simulink model "Acc_Interface"  (R2024b)
settings: Solver=FixedStepAuto  StartTime=0.0  StopTime=inf  FixedStep=5e-3  RelTol=1e-3
InitFcn:
  | %run('config.m');
libraries: arduinolib x2
settings Model: ExtModeTrigDuration=2  Creator=Marc  LastModifiedBy=Nitesh
settings SolverCC: AutoInsertRateTranBlk=on
settings OptimizationCC: DefaultParameterBehavior=Inlined  GainParamInheritBuiltInType=on  UseFloatMulNetSlope=on  InlineInvariantSignals=on  EnhancedBackFolding=on  PassReuseOutputArgsAs=Individual arguments  ZeroExternalMemoryAtStartup=off  ZeroInternalMemoryAtStartup=off  EfficientFloat2IntCast=on  MaxStackSize=64  OptimizeBlockOrder=speed  DifferentSizesBufferReuse=on  OptimizationCustomize=off  EfficientTunableParamExpr=on
settings DebuggingCC: SaveWithParameterizedLinksMsg=none  UnderspecifiedInitializationDetection=Classic  MergeDetectMultiDrivingBlocksExec=none  SignalResolutionControl=TryResolveAllWithWarning  ParameterTunabilityLossMsg=error
settings HardwareCC: ProdBitPerPointer=32  ProdBitPerSizeT=32  ProdBitPerPtrDiffT=32  ProdLargestAtomicInteger=Long  ProdLargestAtomicFloat=Double  ProdWordSize=32  ProdHWDeviceType=ARM Compatible->ARM Cortex  TargetIntDivRoundTo=Zero  TargetEndianess=LittleEndian  TargetHWDeviceType=Custom Processor->Custom Processor  ProdEqTarget=off  UseEmbeddedCoderFeatures=off
settings ModelReferenceCC: PropagateSignalLabelsOutOfModel=off
settings RTWCC: Description=Embedded Coder  SystemTargetFile=ert.tlc  HardwareBoard=ESP32-WROOM(Arduino Compatible)  TLCOptions="-aInlineSetEventsForThisBaseRateFcn=TLC_FALSE -aSuppressMultiTaskScheduler=TLC_FALSE  -aRateBasedStepFcn=0"  TemplateMakefile=ert_default_tmf  Toolchain=ESP32  BuildConfiguration=Faster Runs
settings CodeAppCC: ForceParamTrailComments=on  IgnoreCustomStorageClasses=off  OperatorAnnotations=on  SimulinkDataObjDesc=on  SFDataObjDesc=on  InsertBlockDesc=on
settings ERTTargetCC: SupportNonFinite=off  SupportContinuousTime=on  SupportNonInlinedSFcns=on  SupportVariableSizeSignals=on  ExtModeTransport=3  ExtModeStaticAlloc=on  ExtModeAutomaticAllocSize=off  ExtModeStaticAllocSize=65536  ExtModeMexFile=ext_xcp  ExtModeIntrfLevel=Level2 - Open  InlinedParameterPlacement=Hierarchical

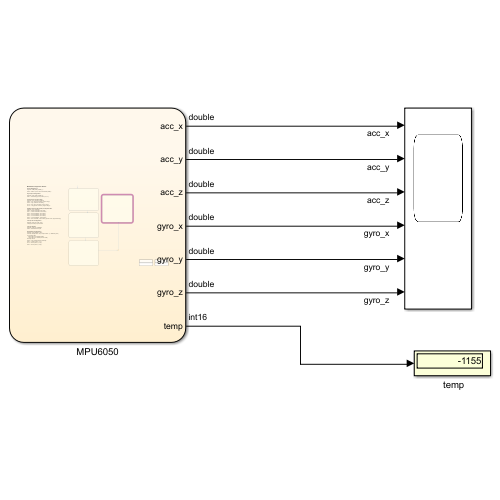
[thumbnail: Simulink's stored preview of the top-level diagram]
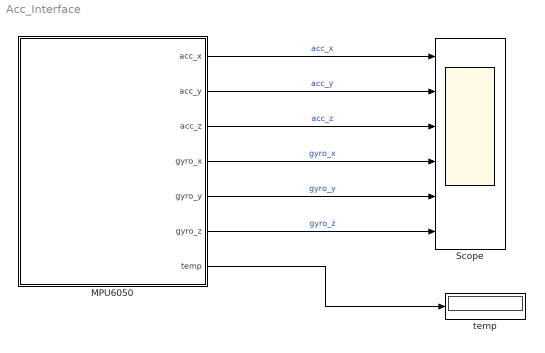
== system Acc_Interface ==
  " temp" : Display
  MPU6050 : Stateflow chart  TreatAsAtomicUnit=on
  Scope : Scope  NumInputPorts=6
  wires:
  MPU6050/1(acc_x) -> Scope/1  "acc_x"
  MPU6050/2(acc_y) -> Scope/2  "acc_y"
  MPU6050/3(acc_z) -> Scope/3  "acc_z"
  MPU6050/7(temp) -> " temp"/1
  MPU6050/4(gyro_x) -> Scope/4  "gyro_x"
  MPU6050/5(gyro_y) -> Scope/5  "gyro_y"
  MPU6050/6(gyro_z) -> Scope/6  "gyro_z"

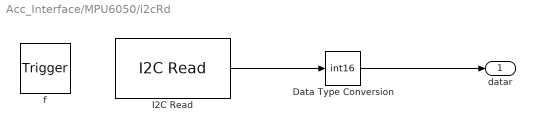
== system Acc_Interface/MPU6050/i2cRd ==
  f : TriggerPort  TriggerType=function-call  VariantControl=Variant  SampleTime=inf
      settings: CopyFcn=Stateflow.SLINSF.SimulinkMan.removeBlockPreDeleteFcn  PreDeleteFcn=Stateflow.SLINSF.SimulinkMan.unsafePredeleteFcn
  Data Type Conversion : DataTypeConversion  OutDataTypeStr=int16  SaturateOnIntegerOverflow=off  RndMeth=Floor
  I2C Read : arduinolib/I2C Read  I2CModule=0  Mode=Master  SlaveAddress=hex2dec( '68' )  SlaveByteOrder=BigEndian  Direction=Receiver  RegisterAddressMode=on  RegisterAddress=hex2dec( '3b' )  SlaveDataType=uint16  DataLength=7  NoAck=off  RepeatedStart=off  OutputStatus=off  blockPlatform=arduino  SampleTime=-1
      settings: SourceProductName=Common
  datar : Outport  Unit=1  VectorParamsAs1DForOutWhenUnconnected=off
  wires:
  I2C Read/1 -> Data Type Conversion/1
  Data Type Conversion/1 -> datar/1

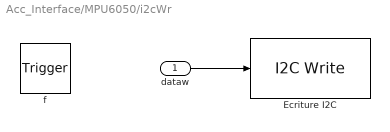
== system Acc_Interface/MPU6050/i2cWr ==
  dataw : Inport  OutDataTypeStr=uint16  Unit=1  PortDimensions=1
  f : TriggerPort  TriggerType=function-call  VariantControl=Variant  SampleTime=-1
      settings: CopyFcn=Stateflow.SLINSF.SimulinkMan.removeBlockPreDeleteFcn  PreDeleteFcn=Stateflow.SLINSF.SimulinkMan.unsafePredeleteFcn
  Ecriture I2C : arduinolib/I2C Write  Priority=1  I2CModule=0  Mode=Master  SlaveAddress=hex2dec( '68' )  SlaveByteOrder=BigEndian  Direction=Transmitter  RegisterAddressMode=off  RegisterAddress=hex2dec( '6B' )  SlaveDataType=uint16  DataLength=1  NoAck=off  RepeatedStart=off  OutputStatus=off  blockPlatform=arduino
      settings: SourceProductName=Common
  wires:
  dataw/1 -> Ecriture I2C/1

== stateflow chart Acc_Interface/MPU6050 ==
  note: MPU6050 Configuration Details
      |
      | Power Management :
      | Register: 0x6B (PWR_MGMT_1)
      | 0x00 → Wake up & use internal oscillator (8MHz)
      |
      | Gyroscope Configuration:
      | Register: 0x6C (PWR_MGMT_2)
      | 0x07 → Disable all gyroscope axes (X, Y, Z)
      |
      | Accelerometer Configuration :
      | Register: 0x1C (ACCEL_CONFIG)
      | 0x00 → ±2g (highest sensitivity, lowest range)
      | 0x08 → ±4g (moderate sensitivity)
      | 0x10 → ±8g (lower sensitivity, higher range)
      | 0x18 → ±16g (lowest sensitivity, highest range)
      |
      | Digital Low-Pass Filter (DLPF) and Update Rate:
      | Register: 0x1A (CONFIG)
      | 0x00 → 260Hz bandwidth, 0ms delay
      | 0x01 → 184Hz bandwidth, 2.0ms delay
      | 0x02 → 94Hz bandwidth, 3.0ms delay
      | 0x03 → 44Hz bandwidth, 4.9ms delay
      | 0x04 → 21Hz bandwidth, 8.5ms delay
      | 0x05 → 10Hz bandwidth, 13.8ms delay
      | 0x06 → 5Hz bandwidth, 19.0ms delay (lowest noise, highest filtering)
      |
      | Interrupt Pin Configuration:
      | Register: 0x37 (INT_PIN_CFG)
      | Configures interrupt pin behavior
      |
      | Interrupt Enable:
      | Register: 0x38 (INT_ENABLE)
      | 0x00 → Disable all interrupts
      |
      | Sample Rate Configuration:
      | Register: 0x19 (SMPLRT_DIV)
      | Formula: Sample Rate = Gyro Output Rate / (1 + SMPLRT_DIV)
      | Gyro Output Rate:
      | - 8kHz if DLPF is disabled (0x00)
      | - 1kHz if DLPF is enabled (0x01 to 0x06)
      | Example values:
      | 0x00 → 1kHz (default if DLPF enabled)
      | 0x07 → 125Hz (1kHz / (1+7))
      | 0x13 → 50Hz (1kHz / (1+19))
      | 0x27 → 25Hz (1kHz / (1+39))
  note: initialisation
      | en:
      | % -------------- Power Management --------------
      | i2cWr(uint16(hex2dec('6B00'))); % Power on
      | % Check if Gyroscope should be disabled
      | if ~ENABLE_GYRO
      |     i2cWr(uint16(hex2dec('6C07'))); % Disable Gyroscope
      | else
      |     i2cWr(uint16(hex2dec('6C00'))); % Enable Gyroscope
      | end
      | % -------------- Accelerometer Configuration --------------
      | switch ACCEL_RANGE
      |     case uint8(2)
      |         i2cWr(uint16(0x1C00));
      |         scale_factor = 16384;  % ±2g
      |     case uint8(4)
      |         i2cWr(uint16(0x1C08));
      |         scale_factor = 8192;   % ±4g
      |     case uint8(8)
      |         i2cWr(uint16(0x1C10));
      |         scale_factor = 4096;   % ±8g
      |     case uint8(16)
      |         i2cWr(uint16(0x1C18));
      |         scale_factor = 2048;   % ±16g
      |     otherwise
      |         error('Invalid Accelerometer Range');
      | end
      | % -------------- Digital Low-Pass Filter --------------
      | if DLPF_SETTING >= 0 && DLPF_SETTING <= 6
      |     i2cWr(uint16(0x1A00) + uint16(DLPF_SETTING));
      | else
      |     error('Invalid DLPF setting');
      | end
      | % -------------- Sampling Configuration --------------
      | % Ensure SAMPLE_RATE_DIV is uint8
      | i2cWr(bitor(0x1900, uint16(uint8(SAMPLE_RATE_DIV))));
      | % -------------- Interrupts --------------
      | i2cWr(uint16(hex2dec('3710'))); % Interrupt pin setup
      | i2cWr(uint16(hex2dec('3800'))); % Disable interrupts
      | disp('MPU6050 Initialization Completed.');
  state initialisation
    en:
    % -------------- Power Management --------------
    i2cWr(uint16(hex2dec('6B00'))); % Power on
    % Check if Gyroscope should be disabled
    if ~ENABLE_GYRO
    i2cWr(uint16(hex2dec('6C07'))); % Disable Gyroscope
    else
    i2cWr(uint16(hex2dec('6C00'))); % Enable Gyroscope
    end
    % -------------- Digital Low-Pass Filter --------------
    if DLPF_SETTING >= 0 && DLPF_SETTING <= 6
    i2cWr(uint16(0x1A00) + uint16(DLPF_SETTING));
    else
    error('Invalid DLPF setting');
    end
  state MPU_Running
    during:
    % Read raw data from MPU6050
    val = i2cRd;
    % Extract acceleration values (X, Y, Z)
    raw_acc_x=val(1);
    raw_acc_y=val(2);
    raw_acc_z=val(3);
    temp = (double(val(4))/340.0) +36.53;
    raw_gryo_x = val(5);
    raw_gryo_y = val(6);
    raw_gryo_z = val(7);
    %
    acc_x = double(raw_acc_x) / double(acc_scale_factor);
    acc_y = double(raw_acc_y) / double(acc_scale_factor);
    acc_z = double(raw_acc_z) / double(acc_scale_factor);
    %
    gyro_x = double(raw_gryo_x) / double(gyro_scale_factor);
    gyro_y = double(raw_gryo_y) / double(gyro_scale_factor);
    gyro_z = double(raw_gryo_z) / double(gyro_scale_factor);
  state Accelerometer_Configuration
    en:
    switch ACCEL_RANGE
    case uint8(2)
    i2cWr(uint16(0x1C00));
    acc_scale_factor = 16384;  % ±2g
    case uint8(4)
    i2cWr(uint16(0x1C08));
    acc_scale_factor = 8192;   % ±4g
    case uint8(8)
    i2cWr(uint16(0x1C10));
    acc_scale_factor = 4096;   % ±8g
    case uint8(16)
    i2cWr(uint16(0x1C18));
    acc_scale_factor = 2048;   % ±16g
    otherwise
    error('Invalid Accelerometer Range');
    end
  state Gyro_Configuration
    en:
    switch GYRO_RANGE
    case 250
    i2cWr(uint16(0x1B00));
    gyro_scale_factor = 131;  % ± 250 °/s
    case 500
    i2cWr(uint16(0x1B08));
    gyro_scale_factor = 65.5;   % ± 500 °/s
    case 1000
    i2cWr(uint16(0x1B10));
    gyro_scale_factor = 32.2;   % ± 1000 °/s
    case 2000
    i2cWr(uint16(0x1B18));
    gyro_scale_factor = 16.4;   % ± 2000 °/s
    otherwise
    error('Invalid Gyro Range');
    end
  state i2cWr(dataw) [function]
  state datar = i2cRd [function]
  (default) -> initialisation
  initialisation -> Accelerometer_Configuration
  (junction 108) -> MPU_Running
  Accelerometer_Configuration -> Gyro_Configuration
  Gyro_Configuration -> (junction 108)
  data: dataw function_input uint16 size=1; datar function_output; val local int16 size=7; acc_x output double; acc_y output double; acc_z output double; raw_acc_x local int16; raw_acc_y local int16; raw_acc_z local int16; acc_scale_factor local uint16 =1; ENABLE_GYRO constant double =1; ACCEL_RANGE constant uint8 =4; SAMPLE_RATE_DIV constant double =0; DLPF_SETTING constant double =6; gyro_x output; gyro_y output; gyro_z output; temp output; GYRO_RANGE constant double =250; gyro_scale_factor local double =1; raw_gryo_y local; raw_gryo_z local; raw_gryo_x local
